simulink model "ShuntExcited_model"  (R2024a)
settings: Solver=VariableStepAuto  StartTime=0.0  StopTime=50  RelTol=1e-3
undefined symbols (not defined in the file or in its folder): B2, dt, dT, J2, La2, Lf2, LoadMode, Ra2, Rf2, Ro, SlopeR, Ts, Vp, Vs
libraries: simulink x1
settings Model: Creator=Xuan  LastModifiedBy=admin
settings RTWCC: GPUComputeCapability=3.5

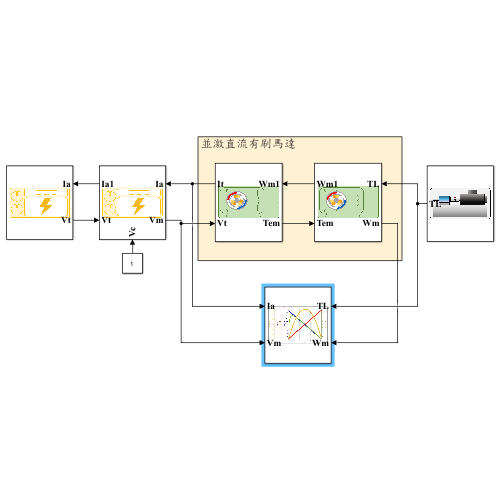
[thumbnail: Simulink's stored preview of the top-level diagram]
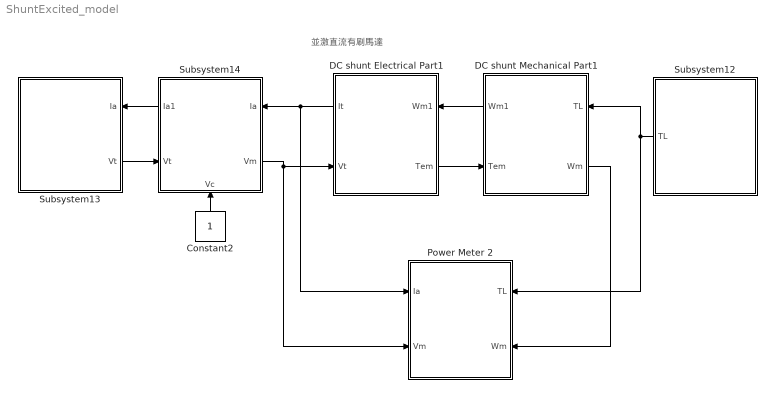
== system ShuntExcited_model ==
  note: 並激直流有刷馬達
  Constant2 : Constant
  DC shunt Electrical Part1 : Subsystem  InitFcn=|
      | La2 = 0.0553;
      | Ra2 = 7.5;
      | Lf2 = 2.4123;
      | Rf2 = 469.75;
      settings: PortSchema="{\"entries\":[{\"content\":{\"sides\":[{\"content\":{\"connectorIds\":[\"Out2\",\"In1\"]},\"type\":\"ConnectorPlacement.EquallySpacedRectSide\",\"uuid\":\"bdb3d079-f1d2-4047-98d5-25417e915914\"},{\"content\":{\"connectorIds\":[\"In2\",\"Out1\"],\"side\":\"RIGHT\"},\"type\":\"ConnectorPlacement.EquallySpacedRectSide\",\"uuid\":\"c8770057-a1bb-4cfe-bc1a-ecb7a24e5078\"},{\"content\":{\"connectorIds\":[],\"side\":\"TOP\"},\"type\":\"ConnectorPlacement.EquallySpacedRectSide\",\"uuid\":\"5ab49577-bec6-4873-973a-4bbd327a98e1\"},{\"content\":{\"connectorIds\":[],\"side\":\"BOTTOM\"},\"type\":\"ConnectorPlacement.EquallySpacedRectSide\",\"uuid\":\"5e523a27-e245-45af-a44d-db5fe349ddd8\"}]},\"type\":\"ConnectorPlacement.EquallySpacedConnector\",\"uuid\":\"511ebc69-457d-4571-bf83-85fa9b668889\"}],\"packageUris\":[\"http://schema.mathworks.com/mf0/Connector/R2020b\"],\"version\":\"1.0\"}"
      mask Display: image('直流並激馬達2.png');
  DC shunt Mechanical Part1 : Subsystem  InitFcn=|
      | J2 = 0.0013;
      | B2 = 0.001;
      settings: PortSchema="{\"entries\":[{\"content\":{\"sides\":[{\"content\":{\"connectorIds\":[\"Out2\",\"In1\"]},\"type\":\"ConnectorPlacement.EquallySpacedRectSide\",\"uuid\":\"bdb3d079-f1d2-4047-98d5-25417e915914\"},{\"content\":{\"connectorIds\":[\"In2\",\"Out1\"],\"side\":\"RIGHT\"},\"type\":\"ConnectorPlacement.EquallySpacedRectSide\",\"uuid\":\"c8770057-a1bb-4cfe-bc1a-ecb7a24e5078\"},{\"content\":{\"connectorIds\":[],\"side\":\"TOP\"},\"type\":\"ConnectorPlacement.EquallySpacedRectSide\",\"uuid\":\"5ab49577-bec6-4873-973a-4bbd327a98e1\"},{\"content\":{\"connectorIds\":[],\"side\":\"BOTTOM\"},\"type\":\"ConnectorPlacement.EquallySpacedRectSide\",\"uuid\":\"5e523a27-e245-45af-a44d-db5fe349ddd8\"}]},\"type\":\"ConnectorPlacement.EquallySpacedConnector\",\"uuid\":\"511ebc69-457d-4571-bf83-85fa9b668889\"}],\"packageUris\":[\"http://schema.mathworks.com/mf0/Connector/R2020b\"],\"version\":\"1.0\"}"
      mask Display: image('直流並激馬達2.png');
  Power Meter 2 : Subsystem  InitFcn=|  StopFcn=|
      InitFcn=|
      | %% ModePlot
      | % PlotMode=1 or 2
      | PlotMode = 2;
      StopFcn=|
      | % %% Data Loading
      | % 
      | % tl2 = out.Tl2;
      | % f2 = size(tl2);
      | % 
      | % % clear datas 
      | % torque2 = 0;
      | % x12 = 0;
      | % y12 = 0; y22 = 0; y32 = 0; y42 = 0; y52 = 0; y62 = 0;
      | % 
      | % switch LoadMode   % mode ( 1:ramp load , 2:stair load )
      | % 
      | %     case 1  
      | % 
      | %         i = 1;
      | %         while 1
      | %             if tl2(i) > 0.01
      | %                s = i;
      | %                break
      | %             end
      | %             i = i+1;
      | %         end
      | %         torque2 = out.Tl2(s:f2(1));
      | %         x12 = out.omega2(s:f2(1));
      | %         % y12 = out.omega2(s:f2(1));
      | %         y22 = out.Eff2(s:f2(1));
      | %         y32 = out.Pin2(s:f2(1));
      | %         y42 = out.Pout2(s:f2(1));
      | %         y52 = out.Vs(s:f2(1));
      | %         y62 = out.Ia2(s:f2(1));
      | %         case 2
      | % 
      | %         tl_pre2 = 0;
      | %         j = 1;
      | %         for i = 1:f2(1)           
      | %             if tl2(i) > tl_pre2
      | %                 torque2(j,1) = tl2(i-1);
      | %                 x12(j,1) = out.omega2((i-1),1);
      | %                 % y12(j,1) = out.omega2((i-1),1);
      | %                 y22(j,1) = out.Eff2((i-1),1);
      | %                 y32(j,1) = out.Pin2((i-1),1);
      | %                 y42(j,1) = out.Pout2((i-1),1);
      | %                 y52(j,1) = out.Vs((i-1),1);
      | %                 y62(j,1) = out.Ia2((i-1),1);
      | %                 j = j+1;
      | %             end
      | %             tl_pre2 = tl2(i);
      | %         end
      | % end
      | % 
      | % %% Plot
      | % % plot TN curve
      | % 
      | % % figure(1);
      | % 
      | % figure(3);
      | % set(gcf, 'Position', [200, 300, 1000, 500]); % [left, bottom, width, height]
      | % clf;
      | % 
      | % % Create empty axis system with 4 y axis by calling:
      | % % handle = maxis(number of axis, y-spacing between outside lines)
      | % h = myaxisc(5,0.10,[0.1,0.1,0.8,0.8]); % Specify position
      | % 
      | % % Call plot and specify y-axis number using method h.p(nr). For creating a
      | % % legend later, we need to assign the handles returned by plot to p.
      | % switch PlotMode
      | % 
      | %     case 1  
      | %         p(1) = plot(h.p(1),x12,torque2,'b','LineWidth',1.2);
      | %         p(2) = plot(h.p(2),x12,y22,'Color',[0.4660 0.6740 0.1880],'LineWidth',1.2);
      | %         p(3) = plot(h.p(3),x12,y62,'Color',[0.3010 0.7450 0.9330],'LineWidth',1.2);
      | %         p(4) = plot(h.p(4),x12,y52,'r','LineWidth',1.2);
      | %         p(5) = plot(h.p(5),x12,y32,'m','LineWidth',1.2);
      | %         print("case1");
      | % 
      | %     case 2
      | %         p(1) = plot(h.p(1),x12,torque2,'b-*','LineWidth',1.1);
      | %         p(2) = plot(h.p(2),x12,y22,'-*','Color',[0.4660 0.6740 0.1880],'LineWidth',1.1);
      | %         p(3) = plot(h.p(3),x12,y62,'-*','Color',[0.3010 0.7450 0.9330],'LineWidth',1.1);
      | %         p(4) = plot(h.p(4),x12,y52,'r-*','LineWidth',1.1);
      | %         p(5) = plot(h.p(5),x12,y32,'m-*','LineWidth',1.1);
      | %         print("case2");
      | % 
      | % end
      | % 
      | % h.autoscale % Automatically Scale Y Axis
      | % 
      | % % Additional methods to modify appearance, scaling and so on:
      | % 
      | % h.autoy(3) % Autoscale only specified y-axis
      | % %h.ylim(3,[95,105]); % Set Y-Limits for axis 3
      | % l = size(torque2);
      | % h.xlim([min(x12),max(x12)+50]);
      | % h.ylim(2,[0,100]); % Set Y-Limits for axis 4
      | % 
      | % h.gridon % Enable grid (use h.gridoff to remove)
      | % 
      | % % Modify the y-Axis Color
      | % h.ycolor(1,'b'); % torque
      | % h.ycolor(2,[0.4660 0.6740 0.1880]); % efficiency
      | % h.ycolor(3,[0.3010 0.7450 0.9330]); % current
      | % h.ycolor(4,'r'); % voltage
      | % h.ycolor(5,'m'); % power in
      | % 
      | % % Add y-Labels
      | % % h.ylabel(1,'Speed (RPM)');
      | % h.ylabel(1, 'TL (Nm)');
      | % h.ylabel(2,'Efficiency (%)');
      | % h.ylabel(3,'Current (A)');
      | % h.ylabel(4,'Voltage (volt)');
      | % h.ylabel(5,'Pin (W)');
      | % 
      | % % Add x-Label
      | % % h.xlabel('TL (Nm)');
      | % h.xlabel('Speed (RPM)');
      | % 
      | % % % Add title
      | % title('TNcurve of Shunt Excited Motor');
      | % set(gca,'FontWeight','bold','FontSize',14);
      | % 
      | % % Change Position of the whole myaxisc-Object
      | % h.position([0.1,0.1,0.8,0.8],0.12); % Position-Vector and Spacing 0.12
      | % 
      | % % Change all font sizes
      | % h.fontsize(10)
      | % 
      | % %% DataSaving
      | % time = out.tout;
      | % powerout2 = out.Pout2;
      | % powerin2 = out.Pin2;
      | % speed2 = out.omega2;
      | % efficiency2 = out.Eff2;
      | % voltage2 = out.Vs;
      | % current2 = out.Ia2;
      | % 
      | % filename = 'Shunt_TNcurve_DataSave.csv';
      | % savedata = [time, powerin2, powerout2, speed2, efficiency2, voltage2, current2];
      | % writematrix(savedata, filename);
      settings: PortSchema="{\"entries\":[{\"content\":{\"sides\":[{\"content\":{\"connectorIds\":[\"In1\",\"In2\"]},\"type\":\"ConnectorPlacement.EquallySpacedRectSide\",\"uuid\":\"e8c36156-32d4-4676-af0d-0891e0773ccb\"},{\"content\":{\"connectorIds\":[\"In3\",\"In4\"],\"side\":\"RIGHT\"},\"type\":\"ConnectorPlacement.EquallySpacedRectSide\",\"uuid\":\"5c876be3-b715-4990-b5f5-1fbda74411c9\"},{\"content\":{\"side\":\"TOP\"},\"type\":\"ConnectorPlacement.EquallySpacedRectSide\",\"uuid\":\"8aaa78a6-3767-49bf-860f-056d8a2101ef\"}]},\"type\":\"ConnectorPlacement.EquallySpacedConnector\",\"uuid\":\"6a38af7a-9eb4-49af-a88b-27cf70b05ead\"}],\"packageUris\":[\"http://schema.mathworks.com/mf0/Connector/R2020b\"],\"version\":\"1.0\"}"
      mask Display: image('TNcurve2.png');
  Subsystem12 : Subsystem  InitFcn=|
      | dt = 0.2;
      | dT = 0.05;
      | Ts = 2;
      | SlopeR = 0.2;
      | % if LoadMode>1.5, then use stair load
      | % if LoadMode<1.5, use linear load
      | LoadMode = 2;
      mask Display: image('主動式動力機2.png');
  Subsystem13 : Subsystem  InitFcn=|
      | Vs = 220;
      | Ro = 0.001;
      settings: PortSchema="{\"entries\":[{\"content\":{\"sides\":[{\"content\":{},\"type\":\"ConnectorPlacement.EquallySpacedRectSide\",\"uuid\":\"717e91a0-288b-4ba5-84da-f262c24688bc\"},{\"content\":{\"connectorIds\":[\"In1\",\"Out1\"],\"side\":\"RIGHT\"},\"type\":\"ConnectorPlacement.EquallySpacedRectSide\",\"uuid\":\"569ee505-38fb-400b-9e45-0fafedafb0f3\"},{\"content\":{\"side\":\"TOP\"},\"type\":\"ConnectorPlacement.EquallySpacedRectSide\",\"uuid\":\"44407c3d-239d-4fc9-b2d2-10ddbad2f525\"}]},\"type\":\"ConnectorPlacement.EquallySpacedConnector\",\"uuid\":\"e894aa65-7991-48d5-91da-50bab94327d3\"}],\"packageUris\":[\"http://schema.mathworks.com/mf0/Connector/R2020b\"],\"version\":\"1.0\"}"
      mask Display: image('直流電源2.png', "center");
  Subsystem14 : Subsystem  InitFcn=Vp = 1;
      settings: PortSchema="{\"entries\":[{\"content\":{\"sides\":[{\"content\":{\"connectorIds\":[\"Out2\",\"In1\"]},\"type\":\"ConnectorPlacement.EquallySpacedRectSide\",\"uuid\":\"717e91a0-288b-4ba5-84da-f262c24688bc\"},{\"content\":{\"connectorIds\":[\"In3\",\"Out1\"],\"side\":\"RIGHT\"},\"type\":\"ConnectorPlacement.EquallySpacedRectSide\",\"uuid\":\"569ee505-38fb-400b-9e45-0fafedafb0f3\"},{\"content\":{\"side\":\"TOP\"},\"type\":\"ConnectorPlacement.EquallySpacedRectSide\",\"uuid\":\"44407c3d-239d-4fc9-b2d2-10ddbad2f525\"},{\"content\":{\"connectorIds\":[\"In2\"],\"side\":\"BOTTOM\"},\"type\":\"ConnectorPlacement.EquallySpacedRectSide\",\"uuid\":\"abc944a0-1837-407a-a5f0-1c34ab870232\"}]},\"type\":\"ConnectorPlacement.EquallySpacedConnector\",\"uuid\":\"e894aa65-7991-48d5-91da-50bab94327d3\"}],\"packageUris\":[\"http://schema.mathworks.com/mf0/Connector/R2020b\"],\"version\":\"1.0\"}"
      mask Display: image('直流電源2.png');
  wires:
  DC shunt Mechanical Part1/1(Wm) -> Power Meter 2/4(Wm)
  DC shunt Electrical Part1/2(It) -> Subsystem14/3(Ia), Power Meter 2/1(Ia)
  DC shunt Mechanical Part1/2(Wm1) -> DC shunt Electrical Part1/2(Wm1)
  DC shunt Electrical Part1/1(Tem) -> DC shunt Mechanical Part1/1(Tem)
  Constant2/1 -> Subsystem14/2(Vc)
  Subsystem12/1(TL) -> DC shunt Mechanical Part1/2(TL), Power Meter 2/3(TL)
  Subsystem14/1(Vm) -> Power Meter 2/2(Vm), DC shunt Electrical Part1/1(Vt)
  Subsystem13/1(Vt) -> Subsystem14/1(Vt)
  Subsystem14/2(Ia1) -> Subsystem13/1(Ia)

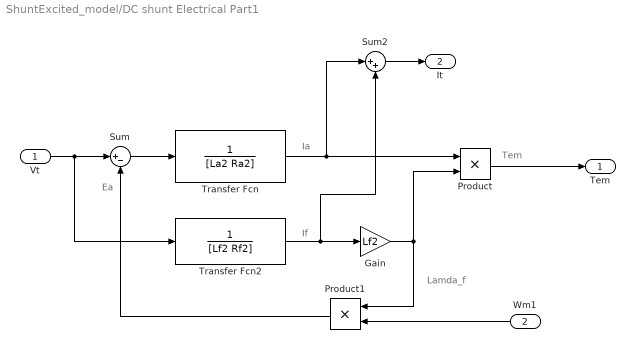
== system ShuntExcited_model/DC shunt Electrical Part1 ==
  note: Ea
  note: Ia
  note: Lamda_f
  note: If
  note: Tem
  Vt : Inport
  Wm1 : Inport  Port=2
  Gain : Gain  Gain=Lf2
  Product : Product
  Product1 : Product
  Sum : Sum  Inputs=|+-
  Sum2 : Sum  Inputs=|++
  Transfer Fcn : TransferFcn  Denominator=[La2 Ra2]
  Transfer Fcn2 : TransferFcn  Denominator=[Lf2 Rf2]
  Tem : Outport
  It : Outport  Port=2
  wires:
  Wm1/1 -> Product1/2
  Product/1 -> Tem/1
  Product1/1 -> Sum/2
  Sum2/1 -> It/1
  Gain/1 -> Product/2, Product1/1
  Sum/1 -> Transfer Fcn/1
  Transfer Fcn/1 -> Sum2/1, Product/1
  Vt/1 -> Transfer Fcn2/1, Sum/1
  Transfer Fcn2/1 -> Sum2/2, Gain/1

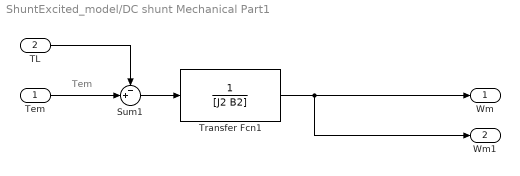
== system ShuntExcited_model/DC shunt Mechanical Part1 ==
  note: Tem
  Tem : Inport
  TL : Inport  Port=2
  Sum1 : Sum  Inputs=-+|
  Transfer Fcn1 : TransferFcn  Denominator=[J2 B2]
  Wm : Outport
  Wm1 : Outport  Port=2
  wires:
  Tem/1 -> Sum1/2
  Transfer Fcn1/1 -> Wm/1, Wm1/1
  TL/1 -> Sum1/1
  Sum1/1 -> Transfer Fcn1/1

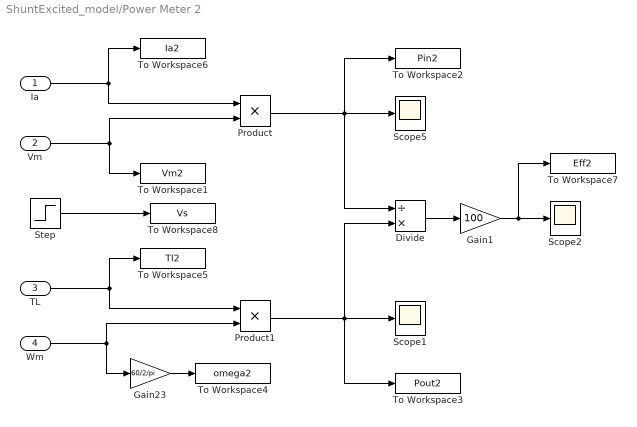
== system ShuntExcited_model/Power Meter 2 ==
  Ia : Inport
  Vm : Inport  Port=2
  TL : Inport  Port=3
  Wm : Inport  Port=4
  Divide : Product  Inputs=/*
  Gain1 : Gain  Gain=100
  Gain23 : Gain  Gain=60/2/pi
  Product : Product
  Product1 : Product
  Scope1 : Scope
  Scope2 : Scope
  Scope5 : Scope
  Step : Step  Time=0.1  After=Vs  SampleTime=0
  To Workspace1 : ToWorkspace  VariableName=Vm2  SampleTime=-1
  To Workspace2 : ToWorkspace  VariableName=Pin2  SampleTime=-1
  To Workspace3 : ToWorkspace  VariableName=Pout2  SampleTime=-1
  To Workspace4 : ToWorkspace  VariableName=omega2  SampleTime=-1
  To Workspace5 : ToWorkspace  VariableName=Tl2  SampleTime=-1
  To Workspace6 : ToWorkspace  VariableName=Ia2  SampleTime=-1
  To Workspace7 : ToWorkspace  VariableName=Eff2  SampleTime=-1
  To Workspace8 : ToWorkspace  VariableName=Vs  SampleTime=-1
  wires:
  Ia/1 -> Product/1, To Workspace6/1
  Vm/1 -> To Workspace1/1, Product/2
  Product/1 -> Divide/1, Scope5/1, To Workspace2/1
  Product1/1 -> Scope1/1, To Workspace3/1, Divide/2
  TL/1 -> To Workspace5/1, Product1/1
  Wm/1 -> Product1/2, Gain23/1
  Gain23/1 -> To Workspace4/1
  Divide/1 -> Gain1/1
  Gain1/1 -> To Workspace7/1, Scope2/1
  Step/1 -> To Workspace8/1

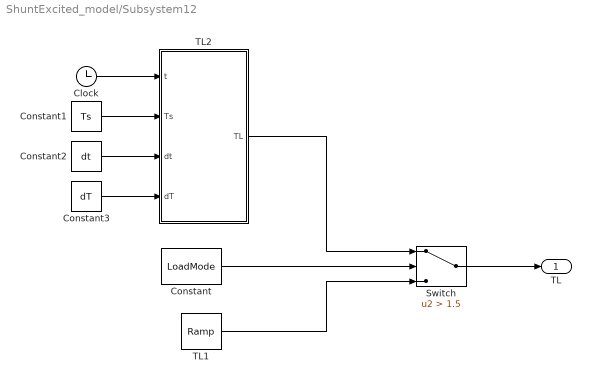
== system ShuntExcited_model/Subsystem12 ==
  Clock : Clock
  Constant : Constant  Value=LoadMode
  Constant1 : Constant  Value=Ts
  Constant2 : Constant  Value=dt  SampleTime=dT
  Constant3 : Constant  Value=dT
  Switch : Switch  Criteria=u2 > Threshold  Threshold=1.5  SaturateOnIntegerOverflow=off  InputSameDT=off
  TL1 : simulink/Sources/Ramp  slope=SlopeR  start=Ts  InitialOutput=0
  TL2 : MATLAB Function  TreatAsAtomicUnit=on
  TL : Outport
  wires:
  Constant2/1 -> TL2/3(dt)
  Constant3/1 -> TL2/4(dT)
  Clock/1 -> TL2/1(t)
  Constant1/1 -> TL2/2(Ts)
  Switch/1 -> TL/1
  Constant/1 -> Switch/2
  TL2/1(TL) -> Switch/1
  TL1/1 -> Switch/3

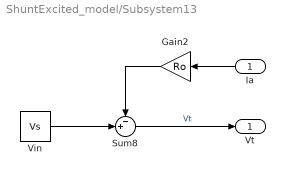
== system ShuntExcited_model/Subsystem13 ==
  Ia : Inport
  Gain2 : Gain  Gain=Ro
  Sum8 : Sum  Inputs=-+|
  Vin : Constant  Value=Vs
  Vt : Outport
  wires:
  Gain2/1 -> Sum8/1
  Sum8/1 -> Vt/1  "Vt"
  Vin/1 -> Sum8/2
  Ia/1 -> Gain2/1

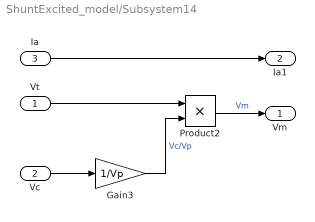
== system ShuntExcited_model/Subsystem14 ==
  Vt : Inport
  Vc : Inport  Port=2
  Ia : Inport  Port=3
  Gain3 : Gain  Gain=1/Vp
  Product2 : Product
  Vm : Outport
  Ia1 : Outport  Port=2
  wires:
  Ia/1 -> Ia1/1
  Vc/1 -> Gain3/1
  Vt/1 -> Product2/1
  Product2/1 -> Vm/1  "Vm"
  Gain3/1 -> Product2/2  "Vc/Vp"

== matlab function ShuntExcited_model/Subsystem12/TL2 ==
  data: t input; Ts input; TL output; dt input; dT input
function TL = fcn(t, Ts, dt, dT)

if t >= Ts
        TL = dT * fix((t-Ts)/dt);
else
    TL = 0;
end
